simulink model "PubIfDecisionLSM_MDL"  (R2020b)
settings: configuration reference "DspaceConfig" (kept outside this file)
PostLoadFcn:
  | if any(exist('dsrtsu_mdlpostloadfcn', 'file') ~= 0), dsrtsu_mdlpostloadfcn('Execute', bdroot); end
InitFcn:
  | , if any(exist('rtifpga_mdlclblib', 'file') ~= 0), rtifpga_mdlclblib('Init', bdroot); end,
  | , if any(exist('dsmpb_private', 'file') ~= 0), dsmpb_private('dsmpb_mdlclblib', 'Init', bdroot); end,
values from neighbouring files (symbols this model uses):
  P_LSM_ALC_Enable = 0.0    [LSM_Parameter.sldd]
  P_LSM_AwayEdge_offset = 0.1    [LSM_Parameter.sldd]
  P_LSM_CentValidErr = 1.0    [LSM_Parameter.sldd]
  P_LSM_DOP_C0_EN_Limit = 0.8    [LSM_Parameter.sldd]
  P_LSM_DOP_C0_out_Limit = 2.0    [LSM_Parameter.sldd]
  P_LSM_DOP_C1_EN_Limit : value not decoded    [LSM_Parameter.sldd]
  P_LSM_DOP_C1_out_Limit : value not decoded    [LSM_Parameter.sldd]
  P_LSM_DOP_C1AndC2_Lim_X : value not decoded    [LSM_Parameter.sldd]
  P_LSM_DOP_C2_EN_Limit : value not decoded    [LSM_Parameter.sldd]
  P_LSM_DOP_C2_out_Limit : value not decoded    [LSM_Parameter.sldd]
  P_LSM_DOP_In_Pre2Dop_Dis = 1.0    [LSM_Parameter.sldd]
  P_LSM_DOP_Out_Pre2Dop_Dis = 2.0    [LSM_Parameter.sldd]
  P_LSM_DOP_PreDis_X : value not decoded    [LSM_Parameter.sldd]
  P_LSM_DOP_PreDis_Y : value not decoded    [LSM_Parameter.sldd]
  P_LSM_DOPEnableSW = 1.0    [LSM_Parameter.sldd]
  P_LSM_DOPValid_CheckTime = 0.06    [LSM_Parameter.sldd]
  P_LSM_DoubleLine_Curr2Cent_Dislimit = 0.5    [LSM_Parameter.sldd]
  P_LSM_DoubleLine_Dop2Cent_Dislimit = 0.5    [LSM_Parameter.sldd]
  P_LSM_DoubleLine_DOPOut_C1 : value not decoded    [LSM_Parameter.sldd]
  P_LSM_DoubleLine_Pre2Cent_Dislimit = 1.0    [LSM_Parameter.sldd]
  P_LSM_Error_Limit = 0.5    [LSM_Parameter.sldd]
  P_LSM_IFV2CenterAxis = 0.0    [LSM_Parameter.sldd]
  P_LSM_IFV2RearAxis = 0.0    [LSM_Parameter.sldd]
  P_LSM_Line2Edge_limit = 0.5    [LSM_Parameter.sldd]
  P_LSM_Line_Error = 0.1    [LSM_Parameter.sldd]
  P_LSM_LineSTD_Limit = 0.15    [LSM_Parameter.sldd]
  P_LSM_NOH_Switch = 0.0    [LSM_Parameter.sldd]
  P_LSM_OTL_C0_Factor = 1.0    [LSM_Parameter.sldd]
  P_LSM_OTL_C1_Factor = 0.5    [LSM_Parameter.sldd]
  P_LSM_OTL_C2_Factor = 0.5    [LSM_Parameter.sldd]
  P_LSM_Pre2OnlyLineDis = 5.0    [LSM_Parameter.sldd]
  P_LSM_Pre_t = 0.0    [LSM_Parameter.sldd]
  P_LSM_SingleLine_Cent2Edge_Dislimit = 100.0    [LSM_Parameter.sldd]
  P_LSM_SingleLine_Curr2Cent_Dislimit = 0.2    [LSM_Parameter.sldd]
  P_LSM_SingleLine_Dop2Cent_Dislimit = 0.2    [LSM_Parameter.sldd]
  P_LSM_SingleLine_DOPOut_C1 : value not decoded    [LSM_Parameter.sldd]
  P_LSM_SingleLine_Pre2Cent_Dislimit = 0.5    [LSM_Parameter.sldd]
  P_LSM_TJALimitSpd = 60.0    [LSM_Parameter.sldd]
undefined symbols (not defined in the file or in its folder): P_lCS_IFV2CenterAxis, P_LCS_IFV2RearAxis, P_LSM_EntryEdge_offset, P_LSM_EntryLnChngEnSwitch, P_LSM_EntryVanishDis, P_LSM_LinetLostTime, P_LSM_LineWijCal_C12, P_LSM_LineWijCal_C13, P_LSM_MapValid_ErrorSwitch, P_LSM_PosLineLcFac, P_LSM_SpdLim_Stub_Spd, P_LSM_SpdLim_StubLength, P_LSM_SpdTurnAlarm
libraries: simulink x324, TrueDurationTime x11
(part 25 of 25)

== matlab function PubIfDecisionLSM_MDL/Subsystem1/TargetLineCalc_20ms/TargetLineCalc/HWALineCalc ==
  data: HWALineC0K1 input; TJA_Line_State input; HWALineValid output boolean size=1; HWASts input uint8 size=1; HWAStsK1 input uint8 size=1; PathValid input boolean; PathA3 input single; PathA2 input single; PathA1 input single; PathA0 input single; PathRange input; PathLaneAvail input; TJALineValid input; TJALineA3 input; TJALineA2 input; TJALineA1 input; TJALineA0 input; TJALineRange input; LeftOffset_b input boolean size=1; RightOffset_b input boolean size=1; HWALineC3 output single size=1; HWALineC2 output single size=1; HWALineC1 output single size=1; HWALineC0 output single size=1; HWARange output single size=1; dDeltaX input single size=1; dDeltaY input single size=1; CosOfPsi input single size=1; SinOfPsi input single size=1; vRef input single size=1; HWALeLineValid output boolean size=1; HWALeLineC3 output single size=1; HWALeLineC2 output single size=1; HWALeLineC1 output single size=1; HWALeLineC0 output single size=1; HWALeRange output single size=1; HWARiLineValid output boolean size=1; HWARiLineC3 output single size=1; HWARiLineC2 output single size=1; HWARiLineC1 output single size=1; HWARiLineC0 output single size=1; HWARiRange output single size=1; preDyDiff output single size=1; HeadAngDiff output single size=1; Error output boolean size=1; MoveIDK1 input int8 size=1; LockIDK1 input int8; MoveID output int8 size=1; LockID output int8; Lock_counterK1 input uint8; Lock_counter output uint8
function [HWALineValid,HWALineC3,HWALineC2,HWALineC1,HWALineC0,HWARange,...
    HWALeLineValid,HWALeLineC3,HWALeLineC2,HWALeLineC1,HWALeLineC0,HWALeRange,...
    HWARiLineValid,HWARiLineC3,HWARiLineC2,HWARiLineC1,HWARiLineC0,HWARiRange,...
    preDyDiff,HeadAngDiff,Error,MoveID,LockID,Lock_counter] = ...
    LineCalc(HWALineC0K1,TJA_Line_State,HWASts,HWAStsK1,...
    PathValid,PathA3,PathA2,PathA1,PathA0,PathRange,PathLaneAvail,...
    TJALineValid,TJALineA3,TJALineA2,TJALineA1,TJALineA0,TJALineRange,...
    LeftOffset_b,RightOffset_b,dDeltaX,dDeltaY,CosOfPsi,SinOfPsi,vRef,MoveIDK1,LockIDK1,Lock_counterK1)

HWALineValid = false;
HWALineC3 = single(0);
HWALineC2 = single(0);
HWALineC1 = single(0);
HWALineC0 = single(0);
HWARange = single(0);
HWALeLineValid = false;
HWALeLineC3 = single(0);
HWALeLineC2 = single(0);
HWALeLineC1 = single(0);
HWALeLineC0 = single(0);
HWALeRange = single(0);
HWARiLineValid = false;
HWARiLineC3 = single(0);
HWARiLineC2 = single(0);
HWARiLineC1 = single(0);
HWARiLineC0 = single(0);
HWARiRange = single(0);
Error = false;
preDis = single(50);

MoveID = MoveIDK1;
LockID = LockIDK1;
if abs(HWALineC0K1)>4.5
    MoveID = int8(0);
    LockID = int8(0);
end

Lock_counter = max(Lock_counterK1-uint8(1),uint8(0));
if Lock_counter==0
    LockID = int8(0);
end

if (HWASts==1)||(HWASts==7)||(HWASts==0)
    MoveID = int8(0);
end

if HWASts ==1 || HWASts == 2
    HWALineValid = TJALineValid;
    HWALineC3 = TJALineA3;
    HWALineC2 = TJALineA2;
    HWALineC1 = TJALineA1;
    HWALineC0 = TJALineA0;
    HWARange = TJALineRange;
end
if HWASts==3
    MoveID = int8(0);
    if HWAStsK1==5 || HWAStsK1==6
        Lock_counter = uint8(250);
        LockID = int8(0);
    end
    if Lock_counter>0
        if LeftOffset_b
            LockID = LockID + int8(1);
        end
        if RightOffset_b
            LockID = LockID - int8(1);
        end
    end
    
    if LockID==1
        HWALineValid = PathValid(3);
        HWALineC3 = PathA3(3);
        HWALineC2 = PathA2(3);
        HWALineC1 = PathA1(3);
        HWALineC0 = PathA0(3);
        HWARange = PathRange(3);
        
        HWALeLineValid = PathValid(2);
        HWALeLineC3 = PathA3(2);
        HWALeLineC2 = PathA2(2);
        HWALeLineC1 = PathA1(2);
        HWALeLineC0 = PathA0(2);
        HWALeRange = PathRange(2);
        
        HWARiLineValid = PathValid(3);
        HWARiLineC3 = PathA3(3);
        HWARiLineC2 = PathA2(3);
        HWARiLineC1 = PathA1(3);
        HWARiLineC0 = PathA0(3);
        HWARiRange = PathRange(3);
        
    elseif LockID==-1
        HWALineValid = PathValid(1);
        HWALineC3 = PathA3(1);
        HWALineC2 = PathA2(1);
        HWALineC1 = PathA1(1);
        HWALineC0 = PathA0(1);
        HWARange = PathRange(1);
        
        HWALeLineValid = PathValid(1);
        HWALeLineC3 = PathA3(1);
        HWALeLineC2 = PathA2(1);
        HWALeLineC1 = PathA1(1);
        HWALeLineC0 = PathA0(1);
        HWALeRange = PathRange(1);
        
        HWARiLineValid = PathValid(2);
        HWARiLineC3 = PathA3(2);
        HWARiLineC2 = PathA2(2);
        HWARiLineC1 = PathA1(2);
        HWARiLineC0 = PathA0(2);
        HWARiRange = PathRange(2);
    elseif LockID==0
        
        HWALineValid = TJALineValid;
        HWALineC3 = TJALineA3;
        HWALineC2 = TJALineA2;
        HWALineC1 = TJALineA1;
        HWALineC0 = TJALineA0;
        HWARange = TJALineRange;
        
        if PathLaneAvail(1)&&(TJA_Line_State==1)&&(PathA0(1)<4.5)
            HWALeLineValid = PathValid(1);
            HWALeLineC3 = PathA3(1);
            HWALeLineC2 = PathA2(1);
            HWALeLineC1 = PathA1(1);
            HWALeLineC0 = PathA0(1);
            HWALeRange = PathRange(1);
        end
        
        if PathLaneAvail(3)&&(TJA_Line_State==1)&&(PathA0(3)>-4.5)
            HWARiLineValid = PathValid(3);
            HWARiLineC3 = PathA3(3);
            HWARiLineC2 = PathA2(3);
            HWARiLineC1 = PathA1(3);
            HWARiLineC0 = PathA0(3);
            HWARiRange = PathRange(3);
        end
    end
end

if HWASts==5
    if HWAStsK1~=5
        MoveID = MoveID - int8(1);
    end
    if LeftOffset_b
        MoveID = MoveID + int8(1);
    end
    if RightOffset_b
        MoveID = MoveID - int8(1);
    end

    if (MoveID>=1)||(MoveID<=-2)
        Error = true;
    end
    if Error==false
        if MoveID==-1
            HWALineValid = PathValid(1);
            HWALineC3 = PathA3(1);
            HWALineC2 = PathA2(1);
            HWALineC1 = PathA1(1);
            HWALineC0 = PathA0(1);
            HWARange = PathRange(1);
            
            HWALeLineValid = PathValid(1);
            HWALeLineC3 = PathA3(1);
            HWALeLineC2 = PathA2(1);
            HWALeLineC1 = PathA1(1);
            HWALeLineC0 = PathA0(1);
            HWALeRange = PathRange(1);
            
            HWARiLineValid = PathValid(2);
            HWARiLineC3 = PathA3(2);
            HWARiLineC2 = PathA2(2);
            HWARiLineC1 = PathA1(2);
            HWARiLineC0 = PathA0(2);
            HWARiRange = PathRange(2);
        elseif MoveID==0
            
            HWALineValid = PathValid(2);
            HWALineC3 = PathA3(2);
            HWALineC2 = PathA2(2);
            HWALineC1 = PathA1(2);
            HWALineC0 = PathA0(2);
            HWARange = PathRange(2);
            
            if PathLaneAvail(1)&&(TJA_Line_State==1)&&(PathA0(1)<4.5)
                HWALeLineValid = PathValid(1);
                HWALeLineC3 = PathA3(1);
                HWALeLineC2 = PathA2(1);
                HWALeLineC1 = PathA1(1);
                HWALeLineC0 = PathA0(1);
                HWALeRange = PathRange(1);
            end
            
            if PathLaneAvail(3)&&(TJA_Line_State==1)&&(PathA0(3)>-4.5)
                HWARiLineValid = PathValid(3);
                HWARiLineC3 = PathA3(3);
                HWARiLineC2 = PathA2(3);
                HWARiLineC1 = PathA1(3);
                HWARiLineC0 = PathA0(3);
                HWARiRange = PathRange(3);
            end
        end
    end
end
if HWASts==6
    if HWAStsK1~=6
        MoveID = MoveID + int8(1);
    end
    if LeftOffset_b
        MoveID = MoveID + int8(1);
    end
    if RightOffset_b
        MoveID = MoveID - int8(1);
    end

    if (MoveID>=2)||(MoveID<=-1)
        Error = true;
    end
    if Error==false
        if MoveID==1
            HWALineValid = PathValid(3);
            HWALineC3 = PathA3(3);
            HWALineC2 = PathA2(3);
            HWALineC1 = PathA1(3);
            HWALineC0 = PathA0(3);
            HWARange = PathRange(3);
            
            HWALeLineValid = PathValid(2);
            HWALeLineC3 = PathA3(2);
            HWALeLineC2 = PathA2(2);
            HWALeLineC1 = PathA1(2);
            HWALeLineC0 = PathA0(2);
            HWALeRange = PathRange(2);
            
            HWARiLineValid = PathValid(3);
            HWARiLineC3 = PathA3(3);
            HWARiLineC2 = PathA2(3);
            HWARiLineC1 = PathA1(3);
            HWARiLineC0 = PathA0(3);
            HWARiRange = PathRange(3);
            
        elseif MoveID==0
            
            HWALineValid = PathValid(2);
            HWALineC3 = PathA3(2);
            HWALineC2 = PathA2(2);
            HWALineC1 = PathA1(2);
            HWALineC0 = PathA0(2);
            HWARange = PathRange(2);
            
            if PathLaneAvail(1)&&(TJA_Line_State==1)&&(PathA0(1)<4.5)
                HWALeLineValid = PathValid(1);
                HWALeLineC3 = PathA3(1);
                HWALeLineC2 = PathA2(1);
                HWALeLineC1 = PathA1(1);
                HWALeLineC0 = PathA0(1);
                HWALeRange = PathRange(1);
            end
            
            if PathLaneAvail(3)&&(TJA_Line_State==1)&&(PathA0(3)>-4.5)
                HWARiLineValid = PathValid(3);
                HWARiLineC3 = PathA3(3);
                HWARiLineC2 = PathA2(3);
                HWARiLineC1 = PathA1(3);
                HWARiLineC0 = PathA0(3);
                HWARiRange = PathRange(3);
            end
        end
    end
end


%% Double Line Lost
t_Dist = max(single(15),vRef*1.8);
x = [0.05*t_Dist;0.3*t_Dist;0.6*t_Dist;t_Dist];
t_dx = x-dDeltaX;
Y_Tar = HWALineC3*x.^3 + HWALineC2*x.^2 + HWALineC1*x + HWALineC0;
dy_Tar = Y_Tar-dDeltaY;
TmpX = t_dx*CosOfPsi+dy_Tar*SinOfPsi;
TmpY = -t_dx*SinOfPsi+dy_Tar*CosOfPsi;
[~,~,HeadAng_Error,preDyDiff] = pl(TmpX,TmpY);
HeadAngDiff = atan(HeadAng_Error)*57.3;
% xOffset = single(2.1);
%
% t_dyDiff = HWALineA3*xOffset^3 + HWALineA2*xOffset^2 + HWALineA1*xOffset + HWALineA0;
% t_A1 = 3*HWALineA3*xOffset^2 + 2*HWALineA2*xOffset + HWALineA1;
% dyDiff = t_dyDiff/sqrt(single(1) + t_A1^2);
